simulink model "model_task1"  (R2025b)
settings: Solver=FixedStepAuto  StartTime=0.0  StopTime=60  FixedStep=0.01  RelTol=1e-3
settings Model: Creator=chris  LastModifiedBy=chris

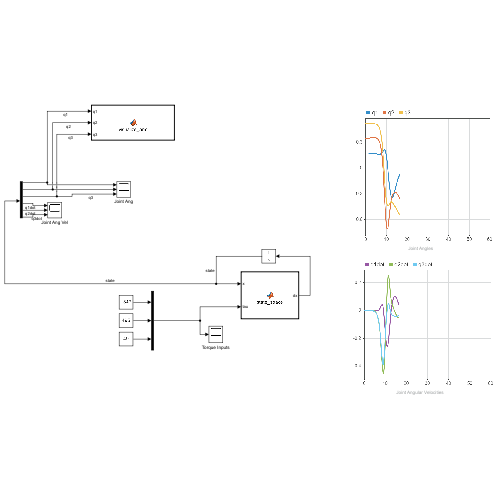
[thumbnail: Simulink's stored preview of the top-level diagram]
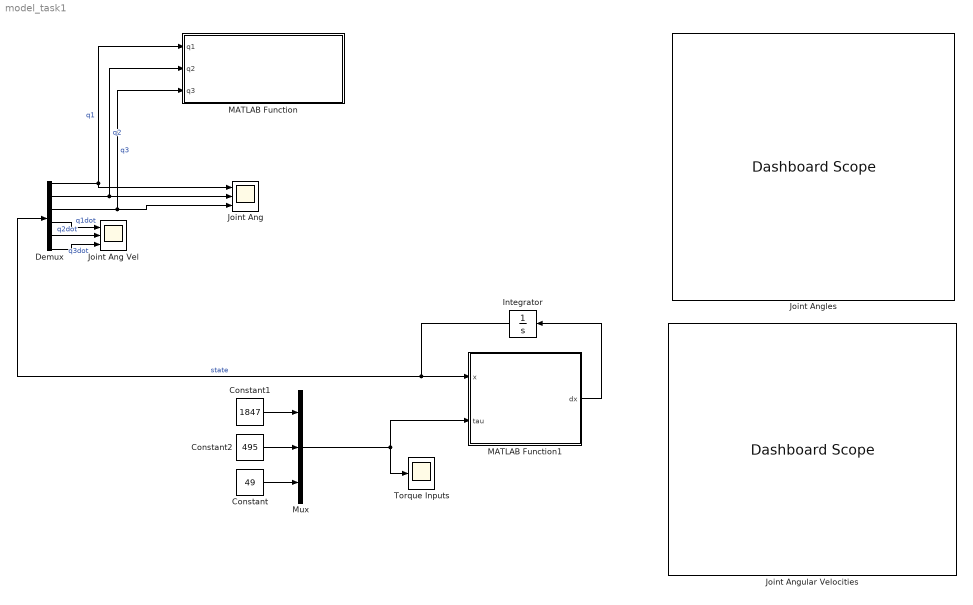
== system model_task1 ==
  Constant : Constant  Value=49
  Constant1 : Constant  Value=1847
  Constant2 : Constant  Value=495
  Demux : Demux  Outputs=6
  Integrator : Integrator  InitialCondition=[10; 20; 30; 0; 0; 0] * (pi/180)
  Joint Ang : Scope  NumInputPorts=3
      settings: ActiveDisplayYMinimum=-0.87065533609721046  ActiveDisplayYMaximum=0.67851589912002208
  Joint Ang Vel : Scope  NumInputPorts=3
      settings: ActiveDisplayYMinimum=-40.868293902570834  ActiveDisplayYMaximum=38.435338076778358
  Joint Angles : DashboardScope  FontColor=[0.0, 0.0, 0.0]
  Joint Angular Velocities : DashboardScope  FontColor=[0.0, 0.0, 0.0]
  MATLAB Function : MATLAB Function  TreatAsAtomicUnit=on  SystemSampleTime=0.01
  MATLAB Function1 : MATLAB Function  TreatAsAtomicUnit=on
  Mux : Mux  Inputs=3
  Torque Inputs : Scope
      settings: ActiveDisplayYMinimum=-20984.614840974609  ActiveDisplayYMaximum=14328.608369338543  DataLoggingVariableName=ScopeData2
  wires:
  MATLAB Function1/1(dx) -> Integrator/1
  Integrator/1 -> Demux/1, MATLAB Function1/1(x)  "state"
  Demux/1 -> Joint Ang/1, MATLAB Function/1(q1)  "q1"
  Demux/2 -> Joint Ang/2, MATLAB Function/2(q2)  "q2"
  Demux/3 -> MATLAB Function/3(q3), Joint Ang/3  "q3"
  Mux/1 -> MATLAB Function1/2(tau), Torque Inputs/1
  Demux/4 -> Joint Ang Vel/1  "q1dot"
  Demux/5 -> Joint Ang Vel/2  "q2dot"
  Demux/6 -> Joint Ang Vel/3  "q3dot"
  Constant/1 -> Mux/3
  Constant1/1 -> Mux/1
  Constant2/1 -> Mux/2

== matlab function model_task1/MATLAB Function1 ==
  data: dx output; x input; tau input
function dx = state_space(x, tau)
%STATE_SPACE  Computes dx for the Lagrangian EOM — Simulink MATLAB Function block.
%
%   EOM:    M(q)*q'' + C(q,q')*q' + G(q) = tau + tau_friction
%   State:  x  = [q1; q2; q3; q1'; q2'; q3']   (6×1)
%   Output: dx = [q'; M\(tau - C*q' - G + tau_friction)]
%
%   All robot parameters are hardcoded below for Simulink compatibility.

    q  = x(1:3);
    dq = x(4:6);

    q = q(:);
    dq = dq(:);
    tau = tau(:);

    %% ── Robot Parameters ──────────────────────────────────────
    L1=4;   L2=3;   L3=2;        %#ok<NASGU> % link lengths      [m]
    m1=20;  m2=15;  m3=10;                   % link masses       [kg]
    Iz1=0.5; Iz2=0.2; Iz3=0.1;              % planar inertias   [kg·m²]
    lc1=2;  lc2=1.5; lc3=1;                 % CoM distances     [m]
    g=9.81;                                  % gravity           [m/s²]
    b1=200;   b2=150;   b3=100;                    % viscous friction  [N·m·s/rad]

    %% ── Dynamic Terms ─────────────────────────────────────────
    M = mass_matrix(q,  m1,m2,m3, Iz1,Iz2,Iz3, L1,L2, lc1,lc2,lc3);
    C = coriolis_matrix(q, dq, m1,m2,m3, Iz1,Iz2,Iz3, L1,L2, lc1,lc2,lc3);
    G = gravity_vector(q,  m1,m2,m3, g, L1,L2, lc1,lc2,lc3);
    tau_friction = friction(dq, b1,b2,b3);

    %% ── State Derivative ──────────────────────────────────────
    ddq = M \ (tau - C*dq - G + tau_friction);
    dx  = [dq; ddq];
end


% ═══════════════════════════════════════════════════════════════
%  SUB-FUNCTIONS
% ═══════════════════════════════════════════════════════════════

function tau_f = friction(dq, b1, b2, b3)
%FRICTION  Viscous joint friction opposing motion.
%   tau_f = -b .* dq      (negative: always opposes velocity)
    tau_f = -[b1*dq(1); b2*dq(2); b3*dq(3)];
end


function M = mass_matrix(q, m1,m2,m3, Iz1,Iz2,Iz3, L1,L2, lc1,lc2,lc3)
%MASS_MATRIX  3×3 joint-space inertia matrix M(q).
%   M = Σᵢ [ mᵢ·Jvᵢ'·Jvᵢ  +  Izᵢ·Jwᵢ'·Jwᵢ ]
%   Jvᵢ: linear velocity Jacobian of CoM i   (2×3)
%   Jwᵢ: angular velocity Jacobian of link i (1×3) — entry j=1 if j≤i

    q1=q(1); q2=q(2); q3=q(3);
    s1=sin(q1);         c1=cos(q1);
    s12=sin(q1+q2);     c12=cos(q1+q2);
    s123=sin(q1+q2+q3); c123=cos(q1+q2+q3);

    % Linear velocity Jacobians (rows: dx/dqj, dy/dqj)
    Jv1 = [ -lc1*s1,                            0,         0 ;
              lc1*c1,                            0,         0 ];

    Jv2 = [ -L1*s1 - lc2*s12,       -lc2*s12,             0 ;
              L1*c1 + lc2*c12,        lc2*c12,             0 ];

    Jv3 = [ -L1*s1 - L2*s12 - lc3*s123,  -L2*s12 - lc3*s123,  -lc3*s123 ;
              L1*c1 + L2*c12 + lc3*c123,   L2*c12 + lc3*c123,   lc3*c123 ];

    % Angular velocity Jacobians (planar: ωᵢ = sum of all upstream q-dots)
    Jw1 = [1, 0, 0];
    Jw2 = [1, 1, 0];
    Jw3 = [1, 1, 1];

    M = m1*(Jv1'*Jv1) + Iz1*(Jw1'*Jw1) + ...
        m2*(Jv2'*Jv2) + Iz2*(Jw2'*Jw2) + ...
        m3*(Jv3'*Jv3) + Iz3*(Jw3'*Jw3);
end


function C = coriolis_matrix(q, dq, m1,m2,m3, Iz1,Iz2,Iz3, L1,L2, lc1,lc2,lc3)
%CORIOLIS_MATRIX  Coriolis & centrifugal matrix via Christoffel symbols.
%   Γ_ijk = ½(∂M_ij/∂q_k + ∂M_ik/∂q_j − ∂M_jk/∂q_i)
%   C_ij  = Σ_k Γ_ijk · q'_k
%   ∂M/∂q via central-difference numerical differentiation.

    n   = 3;
    h   = 1e-7;
    dMdq = zeros(n, n, n);

    for k = 1:n
        qp = q;  qp(k) = q(k) + h;
        qm = q;  qm(k) = q(k) - h;
        Mp = mass_matrix(qp, m1,m2,m3, Iz1,Iz2,Iz3, L1,L2, lc1,lc2,lc3);
        Mm = mass_matrix(qm, m1,m2,m3, Iz1,Iz2,Iz3, L1,L2, lc1,lc2,lc3);
        dMdq(:,:,k) = (Mp - Mm) / (2*h);
    end

    C = zeros(n, n);
    for i = 1:n
        for j = 1:n
            cij = 0;
            for k = 1:n
                Gamma = 0.5*(dMdq(i,j,k) + dMdq(i,k,j) - dMdq(j,k,i));
                cij   = cij + Gamma * dq(k);
            end
            C(i,j) = cij;
        end
    end
end


function G = gravity_vector(q, m1,m2,m3, g, L1,L2, lc1,lc2,lc3)
%GRAVITY_VECTOR  G(q) = ∂PE/∂q,  PE = Σ mᵢ·g·y_ci
%   y_c1 = lc1·sin(q1)
%   y_c2 = L1·sin(q1)  + lc2·sin(q1+q2)
%   y_c3 = L1·sin(q1)  + L2·sin(q1+q2)  + lc3·sin(q1+q2+q3)

    q1=q(1); q2=q(2); q3=q(3);
    c1   = cos(q1);
    c12  = cos(q1+q2);
    c123 = cos(q1+q2+q3);

    G = zeros(3,1);
    G(1) = g*( m1*lc1*c1 + ...
               m2*(L1*c1  + lc2*c12) + ...
               m3*(L1*c1  + L2*c12  + lc3*c123) );
    G(2) = g*( m2*lc2*c12 + ...
               m3*(L2*c12 + lc3*c123) );
    G(3) = g*( m3*lc3*c123 );
end

== matlab function model_task1/MATLAB Function ==
  data: q1 input; q2 input; q3 input
function visualize_arm(q1, q2, q3)
    % Define link lengths
    L1 = 1.0; L2 = 0.8; L3 = 0.5;


    % Base to Link 1 (Rotation at origin)
    T01 = [cos(q1), -sin(q1), 0;
           sin(q1),  cos(q1), 0;
           0,        0,       1];
       
    % Link 1 to Link 2 (Translate by L1, then rotate by q2)
    T12 = [cos(q2), -sin(q2), L1;
           sin(q2),  cos(q2), 0;
           0,        0,       1];
       
    % Link 2 to Link 3 (Translate by L2, then rotate by q3)
    T23 = [cos(q3), -sin(q3), L2;
           sin(q3),  cos(q3), 0;
           0,        0,       1];

    % 2. Calculate Global Positions
    % Points are defined as [0; 0; 1] in their local frames
    P0 = [0; 0; 1];                     % Base
    P1 = T01 * [0; 0; 1];               % Joint 1
    P2 = T01 * T12 * [0; 0; 1];         % Joint 2
    P3 = T01 * T12 * T23 * [0; 0; 1];   % End Effector (Translate by L3 from P2)
    
    % The end effector tip is L3 away from P3 along its local x-axis
    P_tip = T01 * T12 * T23 * [L3; 0; 1];

    % 3. Extract Coordinates for Plotting
    X = [P0(1), P1(1), P2(1), P3(1), P_tip(1)];
    Y = [P0(2), P1(2), P2(2), P3(2), P_tip(2)];
    
        % 4. Graphics Handling
    persistent h;
    
    if isempty(h)
        figure('Name', '3R Robot - Matrix Kinematics');
        h = plot(X, Y, '-o', 'LineWidth', 2, 'MarkerFaceColor', 'k');
        grid on; axis equal;
        limit = L1 + L2 + L3 + 0.5;
        axis([-limit limit -limit limit]);
    else
        if ~ishandle(h)
            figure('Name', '3R Robot - Matrix Kinematics');
            h = plot(X, Y, '-o', 'LineWidth', 2, 'MarkerFaceColor', 'k');
            grid on; axis equal;
            limit = L1 + L2 + L3 + 0.5;
            axis([-limit limit -limit limit]);
        else
            set(h, 'XData', X, 'YData', Y);
        end
    end
    drawnow;
end
